simulink model "Progetto_1_0"  (R2015b)
settings: Solver=FixedStepDiscrete  SolverMode=SingleTasking  StartTime=0.0  StopTime=1500  FixedStep=1/100  RelTol=1e-3
values from neighbouring files (symbols this model uses):
  End_Time = s*z + l*z + l*x + 10    [Start_1_0.m]
  MASK = [0.111111111111  0.111111111111  0.111111111111; 0.111111111111  0.111111111111  0.111111111111; 0.111111111111  0.111111111111  0.111111111111]    [mask_3x3.mat]    (also in mask_3x3_egual.mat = [0  0  0; 0  1  0; 0  0  0]; mask_3x3_zeros.mat = [0  0  0; 0  0  0; 0  0  0]; mask_5x5.mat = [0.04 0.04 0.04 0.04 0.04 0.04 0.04 0.04 0.04 0.04 0.04 0.04; mask_5x5_egual.mat = [0 0 0 0 0 0 0 0 0 0 0 0 ... (25 elements, 5x5)])
libraries: hdlsllib x3, visionsources x1
settings Model: Creator=danilo  LastModifiedBy=danilo

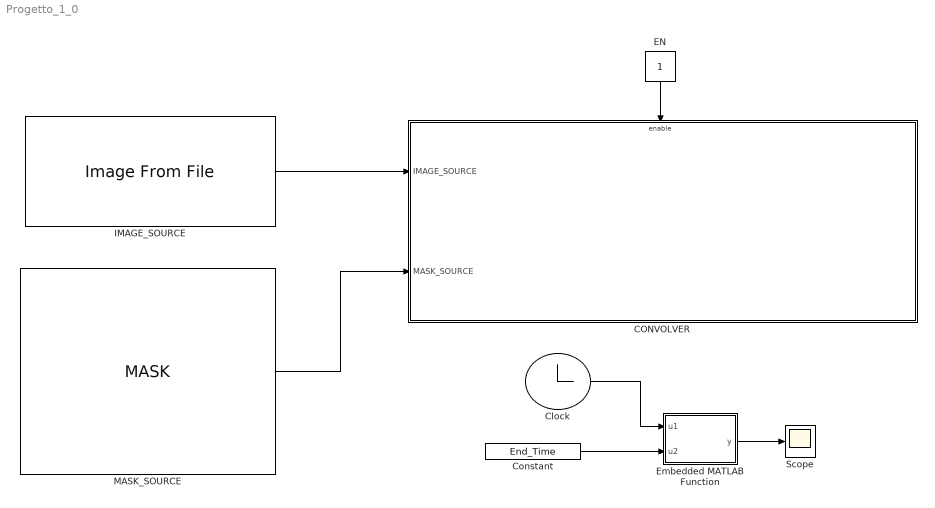
== system Progetto_1_0 ==
  CONVOLVER : Subsystem
  Clock : Clock
  Constant : Constant  Value=End_Time
  EN : Constant
  Embedded MATLAB Function : MATLAB Function  TreatAsAtomicUnit=on
  IMAGE_SOURCE : visionsources/Image From File  Tag=vipblks_nd  FileName=./test_23x10.jpg  imagePorts=One multidimensional signal  Ts=inf  ImageDataType=Inherit from input image  Signed=on  WordLength=16  sdImageDataType=uint(8)  FractionLengthMode=User-defined  FractionLength=15  OutPortLabels=R|G|B
  "MASK_SOURCE " : Constant  Value=MASK
  Scope : Scope
  wires:
  IMAGE_SOURCE/1 -> CONVOLVER/1(IMAGE_SOURCE)
  EN/1 -> CONVOLVER/Enable
  Clock/1 -> Embedded MATLAB Function/1(u1)
  Constant/1 -> Embedded MATLAB Function/2(u2)
  Embedded MATLAB Function/1(y) -> Scope/1
  "MASK_SOURCE "/1 -> CONVOLVER/2(MASK_SOURCE)

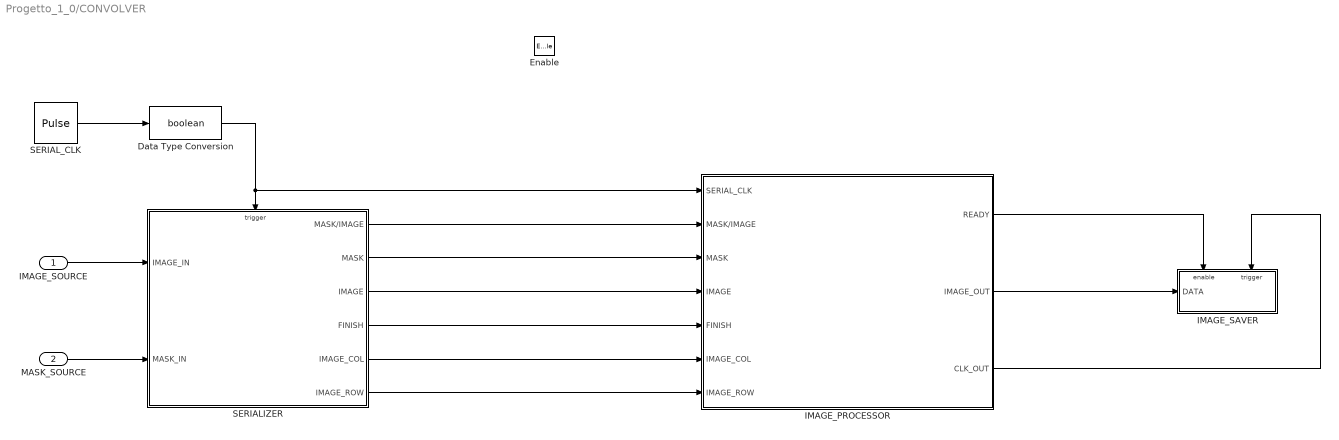
== system Progetto_1_0/CONVOLVER ==
  IMAGE_SOURCE : Inport
  MASK_SOURCE : Inport  Port=2
  Enable : EnablePort
  Data Type Conversion : DataTypeConversion  OutDataTypeStr=boolean
  IMAGE_PROCESSOR : Subsystem
  "IMAGE_SAVER " : Subsystem  TreatAsAtomicUnit=on
  SERIALIZER : Subsystem
  SERIAL_CLK : DiscretePulseGenerator  PulseType=Time based  Period=1  PulseWidth=50
  wires:
  MASK_SOURCE/1 -> SERIALIZER/2(MASK_IN)
  IMAGE_SOURCE/1 -> SERIALIZER/1(IMAGE_IN)
  SERIALIZER/5(IMAGE_COL) -> IMAGE_PROCESSOR/6(IMAGE_COL)
  SERIALIZER/3(IMAGE) -> IMAGE_PROCESSOR/4(IMAGE)
  SERIALIZER/4(FINISH) -> IMAGE_PROCESSOR/5(FINISH)
  SERIAL_CLK/1 -> Data Type Conversion/1
  Data Type Conversion/1 -> IMAGE_PROCESSOR/1(SERIAL_CLK), SERIALIZER/Trigger
  SERIALIZER/2(MASK) -> IMAGE_PROCESSOR/3(MASK)
  SERIALIZER/1(MASK/IMAGE) -> IMAGE_PROCESSOR/2(MASK/IMAGE)
  SERIALIZER/6(IMAGE_ROW) -> IMAGE_PROCESSOR/7(IMAGE_ROW)
  IMAGE_PROCESSOR/2(IMAGE_OUT) -> "IMAGE_SAVER "/1(DATA)
  IMAGE_PROCESSOR/1(READY) -> "IMAGE_SAVER "/Enable
  IMAGE_PROCESSOR/3(CLK_OUT) -> "IMAGE_SAVER "/Trigger

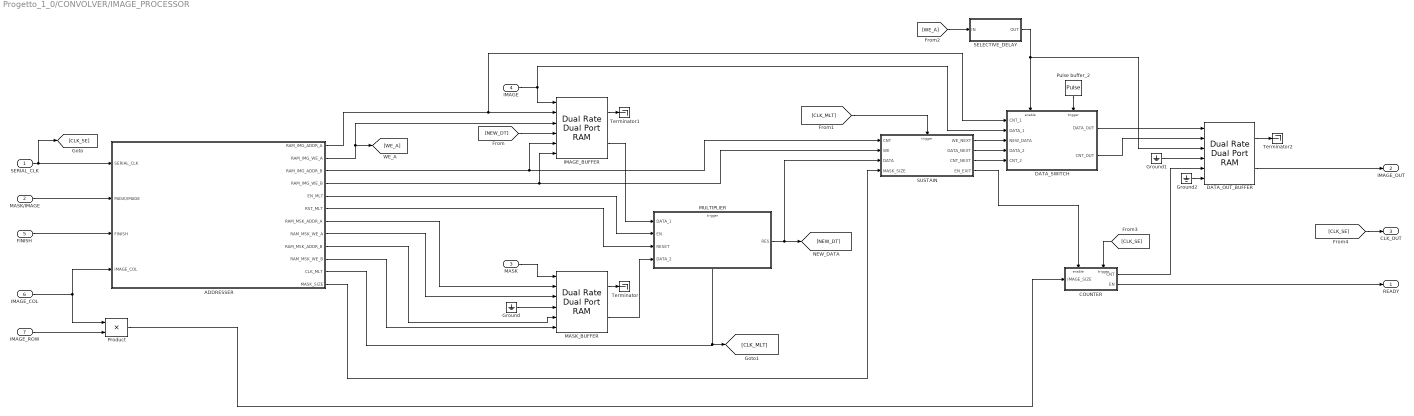
== system Progetto_1_0/CONVOLVER/IMAGE_PROCESSOR ==
  SERIAL_CLK : Inport  OutDataTypeStr=boolean
  MASK/IMAGE : Inport  Port=2  OutDataTypeStr=boolean
  MASK : Inport  Port=3  OutDataTypeStr=double
  IMAGE : Inport  Port=4  OutDataTypeStr=uint8
  FINISH : Inport  Port=5  OutDataTypeStr=boolean
  IMAGE_COL : Inport  Port=6  OutDataTypeStr=double
  IMAGE_ROW : Inport  Port=7  OutDataTypeStr=double
  ADDRESSER : Subsystem  TreatAsAtomicUnit=on
  COUNTER : Subsystem  TreatAsAtomicUnit=on
  DATA_OUT_BUFFER : hdlsllib/HDL Operations/Dual Rate Dual Port RAM  ram_size=16
  DATA_SWITCH : Subsystem  TreatAsAtomicUnit=on
  Ground : Ground
  Ground1 : Ground
  Ground2 : Ground
  IMAGE_BUFFER : hdlsllib/HDL Operations/Dual Rate Dual Port RAM  ram_size=16
  MASK_BUFFER : hdlsllib/HDL Operations/Dual Rate Dual Port RAM  ram_size=16
  MULTIPLIER : Subsystem
  Product : Product
  "Pulse buffer_2 " : DiscretePulseGenerator  PulseType=Time based  Period=1/2  PulseWidth=50
  SELECTIVE_DELAY : Subsystem
  SUSTAIN : Subsystem  TreatAsAtomicUnit=on
  Terminator : Terminator
  Terminator1 : Terminator
  Terminator2 : Terminator
  READY : Outport
  IMAGE_OUT : Outport  Port=2
  CLK_OUT : Outport  Port=3
  wires:
  MASK/IMAGE/1 -> ADDRESSER/2(MASK/IMAGE)
  MASK/1 -> MASK_BUFFER/1
  IMAGE/1 -> IMAGE_BUFFER/1, DATA_SWITCH/2(DATA_1)
  ADDRESSER/3(RAM_IMG_ADDR_B) -> SUSTAIN/1(CNT), IMAGE_BUFFER/5
  ADDRESSER/7(RAM_MSK_ADDR_A) -> MASK_BUFFER/2
  ADDRESSER/8("RAM_MSK_WE_A ") -> MASK_BUFFER/3
  ADDRESSER/9(RAM_MSK_ADDR_B) -> MASK_BUFFER/5
  ADDRESSER/10(RAM_MSK_WE_B) -> MASK_BUFFER/6
  MASK_BUFFER/2 -> MULTIPLIER/4(DATA_2)
  ADDRESSER/5(EN_MLT) -> MULTIPLIER/2(EN)
  ADDRESSER/6(RST_MLT) -> MULTIPLIER/3(RESET)
  MULTIPLIER/1(RES) -> SUSTAIN/3(DATA), [NEW_DT]
  [NEW_DT] -> IMAGE_BUFFER/4
  IMAGE_COL/1 -> Product/1, ADDRESSER/4(IMAGE_COL)
  ADDRESSER/11(CLK_MLT) -> [CLK_MLT], MULTIPLIER/Trigger
  MASK_BUFFER/1 -> Terminator/1
  Ground/1 -> MASK_BUFFER/4
  IMAGE_BUFFER/2 -> MULTIPLIER/1(DATA_1)
  "Pulse buffer_2 "/1 -> DATA_SWITCH/Trigger
  ADDRESSER/2("RAM_IMG_WE_A ") -> [WE_A], IMAGE_BUFFER/3
  SERIAL_CLK/1 -> [CLK_SE], ADDRESSER/1(SERIAL_CLK)
  SUSTAIN/2(DATA_NEXT) -> DATA_SWITCH/4(DATA_2)
  SUSTAIN/1(WE_NEXT) -> DATA_SWITCH/3(NEW_DATA)
  DATA_SWITCH/2(CNT_OUT) -> DATA_OUT_BUFFER/2
  DATA_OUT_BUFFER/2 -> IMAGE_OUT/1
  [WE_A] -> SELECTIVE_DELAY/1(IN)
  SELECTIVE_DELAY/1(OUT) -> DATA_SWITCH/Enable, DATA_OUT_BUFFER/3
  ADDRESSER/1(RAM_IMG_ADDR_A) -> DATA_SWITCH/1(CNT_1), IMAGE_BUFFER/2
  [CLK_SE] -> COUNTER/Trigger
  COUNTER/1(CNT) -> DATA_OUT_BUFFER/5
  FINISH/1 -> ADDRESSER/3(FINISH)
  DATA_SWITCH/1(DATA_OUT) -> DATA_OUT_BUFFER/1
  ADDRESSER/4(RAM_IMG_WE_B) -> SUSTAIN/2(WE), IMAGE_BUFFER/6
  SUSTAIN/3(CNT_NEXT) -> DATA_SWITCH/5(CNT_2)
  SUSTAIN/4(EN_EXIT) -> COUNTER/Enable
  [CLK_MLT] -> SUSTAIN/Trigger
  ADDRESSER/12(MASK_SIZE) -> SUSTAIN/4(MASK_SIZE)
  IMAGE_BUFFER/1 -> Terminator1/1
  Ground1/1 -> DATA_OUT_BUFFER/4
  Ground2/1 -> DATA_OUT_BUFFER/6
  IMAGE_ROW/1 -> Product/2
  Product/1 -> COUNTER/1(IMAGE_SIZE)
  COUNTER/2(EN) -> READY/1
  [CLK_SE] -> CLK_OUT/1
  DATA_OUT_BUFFER/1 -> Terminator2/1

== system Progetto_1_0/CONVOLVER/IMAGE_SAVER  ==
  DATA : Inport
  Enable : EnablePort
  Trigger : TriggerPort
  To Workspace : ToWorkspace  VariableName=simout  SampleTime=-1
      settings: Save2DSignal=2-D array (concatenate along first dimension)
  wires:
  DATA/1 -> To Workspace/1

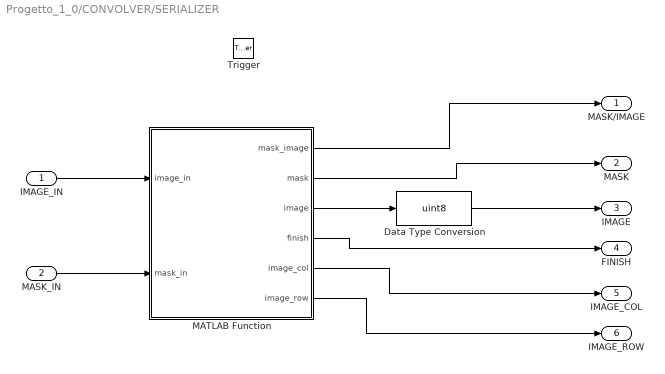
== system Progetto_1_0/CONVOLVER/SERIALIZER ==
  IMAGE_IN : Inport  OutDataTypeStr=uint8
  MASK_IN : Inport  Port=2
  Trigger : TriggerPort  PortDimensions=1
  Data Type Conversion : DataTypeConversion  OutDataTypeStr=uint8
  MATLAB Function : MATLAB Function  TreatAsAtomicUnit=on
  MASK/IMAGE : Outport
  MASK : Outport  Port=2  OutDataTypeStr=double
  IMAGE : Outport  Port=3
  FINISH : Outport  Port=4
  IMAGE_COL : Outport  Port=5  OutDataTypeStr=double
  IMAGE_ROW : Outport  Port=6  OutDataTypeStr=double
  wires:
  IMAGE_IN/1 -> MATLAB Function/1(image_in)
  MASK_IN/1 -> MATLAB Function/2(mask_in)
  MATLAB Function/1(mask_image) -> MASK/IMAGE/1
  MATLAB Function/3(image) -> Data Type Conversion/1
  MATLAB Function/4(finish) -> FINISH/1
  MATLAB Function/2(mask) -> MASK/1
  Data Type Conversion/1 -> IMAGE/1
  MATLAB Function/5(image_col) -> IMAGE_COL/1
  MATLAB Function/6(image_row) -> IMAGE_ROW/1

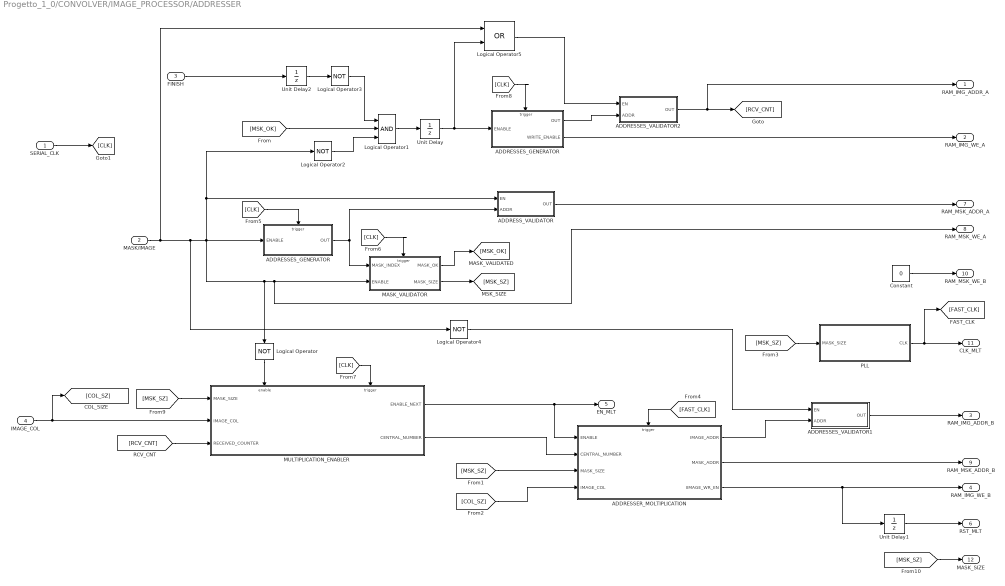
== system Progetto_1_0/CONVOLVER/IMAGE_PROCESSOR/ADDRESSER ==
  SERIAL_CLK : Inport
  MASK/IMAGE : Inport  Port=2
  FINISH : Inport  Port=3
  IMAGE_COL : Inport  Port=4  OutDataTypeStr=double
  ADDRESSER_MOLTIPLICATION : Subsystem  TreatAsAtomicUnit=on
  ADDRESSES_GENERATOR : Subsystem
  "ADDRESSES_GENERATOR " : Subsystem
  ADDRESSES_VALIDATOR1 : Subsystem
  ADDRESSES_VALIDATOR2 : Subsystem
  ADDRESS_VALIDATOR : Subsystem
  Constant : Constant  Value=0  OutDataTypeStr=boolean
  Logical Operator{,2..4} (4 alike) : Logic  Operator=NOT  AllPortsSameDT=off  OutDataTypeStr=boolean
  Logical Operator1 : Logic  Inputs=3  AllPortsSameDT=off  OutDataTypeStr=boolean
  Logical Operator5 : Logic  Operator=OR  AllPortsSameDT=off  OutDataTypeStr=boolean
  MASK_VALIDATOR : Subsystem
  MULTIPLICATION_ENABLER : Subsystem  TreatAsAtomicUnit=on
  PLL : Subsystem  TreatAsAtomicUnit=on
  Unit Delay : UnitDelay  SampleTime=-1
  Unit Delay1 : UnitDelay  SampleTime=-1
  Unit Delay2 : UnitDelay  SampleTime=-1
  RAM_IMG_ADDR_A : Outport
  "RAM_IMG_WE_A " : Outport  Port=2
  RAM_IMG_ADDR_B : Outport  Port=3
  RAM_IMG_WE_B : Outport  Port=4
  EN_MLT : Outport  Port=5
  RST_MLT : Outport  Port=6
  RAM_MSK_ADDR_A : Outport  Port=7  OutDataTypeStr=uint16
  "RAM_MSK_WE_A " : Outport  Port=8
  RAM_MSK_ADDR_B : Outport  Port=9
  RAM_MSK_WE_B : Outport  Port=10
  CLK_MLT : Outport  Port=11
  MASK_SIZE : Outport  Port=12
  wires:
  "ADDRESSES_GENERATOR "/1(OUT) -> ADDRESS_VALIDATOR/2(ADDR), MASK_VALIDATOR/1(MASK_INDEX)
  MASK_VALIDATOR/1(MASK_OK) -> [MSK_OK]
  Logical Operator1/1 -> Unit Delay/1
  Unit Delay/1 -> Logical Operator5/2, ADDRESSES_GENERATOR/1(ENABLE)
  FINISH/1 -> Unit Delay2/1
  ADDRESSES_VALIDATOR1/1(OUT) -> RAM_IMG_ADDR_B/1
  IMAGE_COL/1 -> MULTIPLICATION_ENABLER/2(IMAGE_COL), [COL_SZ]
  [RCV_CNT] -> MULTIPLICATION_ENABLER/3(RECEIVED_COUNTER)
  Logical Operator/1 -> MULTIPLICATION_ENABLER/Enable
  MULTIPLICATION_ENABLER/2(CENTRAL_NUMBER) -> ADDRESSER_MOLTIPLICATION/2(CENTRAL_NUMBER)
  [MSK_SZ] -> ADDRESSER_MOLTIPLICATION/3(MASK_SIZE)
  [COL_SZ] -> ADDRESSER_MOLTIPLICATION/4(IMAGE_COL)
  ADDRESSER_MOLTIPLICATION/1(IMAGE_ADDR) -> ADDRESSES_VALIDATOR1/2(ADDR)
  ADDRESSER_MOLTIPLICATION/2(MASK_ADDR) -> RAM_MSK_ADDR_B/1
  Constant/1 -> RAM_MSK_WE_B/1
  Unit Delay1/1 -> RST_MLT/1
  PLL/1(CLK) -> [FAST_CLK], CLK_MLT/1
  [MSK_SZ] -> PLL/1(MASK_SIZE)
  [FAST_CLK] -> ADDRESSER_MOLTIPLICATION/Trigger
  SERIAL_CLK/1 -> [CLK]
  [CLK] -> "ADDRESSES_GENERATOR "/Trigger
  [CLK] -> MASK_VALIDATOR/Trigger
  [CLK] -> MULTIPLICATION_ENABLER/Trigger
  [CLK] -> ADDRESSES_GENERATOR/Trigger
  ADDRESS_VALIDATOR/1(OUT) -> RAM_MSK_ADDR_A/1
  MASK_VALIDATOR/2(MASK_SIZE) -> [MSK_SZ]
  [MSK_SZ] -> MULTIPLICATION_ENABLER/1(MASK_SIZE)
  Unit Delay2/1 -> Logical Operator3/1
  ADDRESSES_GENERATOR/2(WRITE_ENABLE) -> "RAM_IMG_WE_A "/1
  ADDRESSER_MOLTIPLICATION/3(IIMAGE_WR_EN) -> Unit Delay1/1, RAM_IMG_WE_B/1
  Logical Operator2/1 -> Logical Operator1/3
  [MSK_OK] -> Logical Operator1/2
  Logical Operator3/1 -> Logical Operator1/1
  MULTIPLICATION_ENABLER/1("ENABLE_NEXT ") -> ADDRESSER_MOLTIPLICATION/1(ENABLE), EN_MLT/1
  Logical Operator4/1 -> ADDRESSES_VALIDATOR1/1(EN)
  MASK/IMAGE/1 -> "ADDRESSES_GENERATOR "/1(ENABLE), Logical Operator/1, "RAM_MSK_WE_A "/1, MASK_VALIDATOR/2(ENABLE), ADDRESS_VALIDATOR/1(EN), Logical Operator2/1, Logical Operator4/1, Logical Operator5/1
  ADDRESSES_VALIDATOR2/1(OUT) -> RAM_IMG_ADDR_A/1, [RCV_CNT]
  ADDRESSES_GENERATOR/1(OUT) -> ADDRESSES_VALIDATOR2/2(ADDR)
  Logical Operator5/1 -> ADDRESSES_VALIDATOR2/1(EN)
  [MSK_SZ] -> MASK_SIZE/1

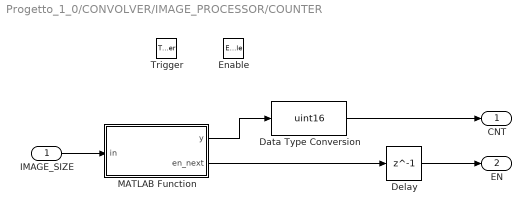
== system Progetto_1_0/CONVOLVER/IMAGE_PROCESSOR/COUNTER ==
  IMAGE_SIZE : Inport
  Enable : EnablePort
  Trigger : TriggerPort
  Data Type Conversion : DataTypeConversion  OutDataTypeStr=uint16
  Delay : Delay  DelayLength=1  InitialCondition=0
  MATLAB Function : MATLAB Function  TreatAsAtomicUnit=on
  CNT : Outport
  EN : Outport  Port=2
  wires:
  MATLAB Function/1(y) -> Data Type Conversion/1
  Data Type Conversion/1 -> CNT/1
  IMAGE_SIZE/1 -> MATLAB Function/1(in)
  MATLAB Function/2(en_next) -> Delay/1
  Delay/1 -> EN/1

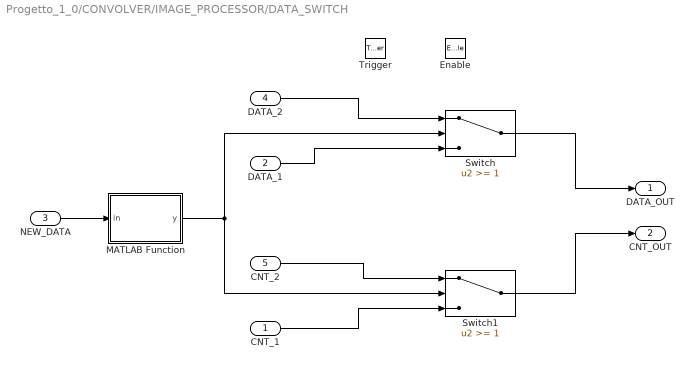
== system Progetto_1_0/CONVOLVER/IMAGE_PROCESSOR/DATA_SWITCH ==
  CNT_1 : Inport
  DATA_1 : Inport  Port=2
  NEW_DATA : Inport  Port=3
  DATA_2 : Inport  Port=4
  CNT_2 : Inport  Port=5
  Enable : EnablePort
  Trigger : TriggerPort
  MATLAB Function : MATLAB Function  TreatAsAtomicUnit=on
  Switch : Switch  Threshold=1
  Switch1 : Switch  Threshold=1
  DATA_OUT : Outport
  CNT_OUT : Outport  Port=2
  wires:
  Switch/1 -> DATA_OUT/1
  DATA_2/1 -> Switch/1
  DATA_1/1 -> Switch/3
  CNT_2/1 -> Switch1/1
  Switch1/1 -> CNT_OUT/1
  CNT_1/1 -> Switch1/3
  NEW_DATA/1 -> MATLAB Function/1(in)
  MATLAB Function/1(y) -> Switch/2, Switch1/2

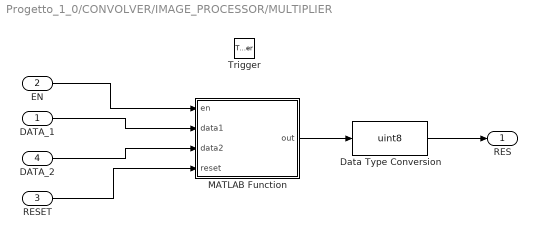
== system Progetto_1_0/CONVOLVER/IMAGE_PROCESSOR/MULTIPLIER ==
  DATA_1 : Inport
  EN : Inport  Port=2
  RESET : Inport  Port=3
  DATA_2 : Inport  Port=4
  Trigger : TriggerPort  PortDimensions=1
  Data Type Conversion : DataTypeConversion  OutDataTypeStr=uint8
  MATLAB Function : MATLAB Function  TreatAsAtomicUnit=on
  RES : Outport
  wires:
  MATLAB Function/1(out) -> Data Type Conversion/1
  EN/1 -> MATLAB Function/1(en)
  DATA_1/1 -> MATLAB Function/2(data1)
  DATA_2/1 -> MATLAB Function/3(data2)
  Data Type Conversion/1 -> RES/1
  RESET/1 -> MATLAB Function/4(reset)

== system Progetto_1_0/CONVOLVER/IMAGE_PROCESSOR/SELECTIVE_DELAY ==
  IN : Inport
  Switch : Switch  Threshold=1
  Unit Delay : UnitDelay  SampleTime=-1
  OUT : Outport
  wires:
  Unit Delay/1 -> Switch/3
  Switch/1 -> OUT/1
  IN/1 -> Unit Delay/1, Switch/1, Switch/2

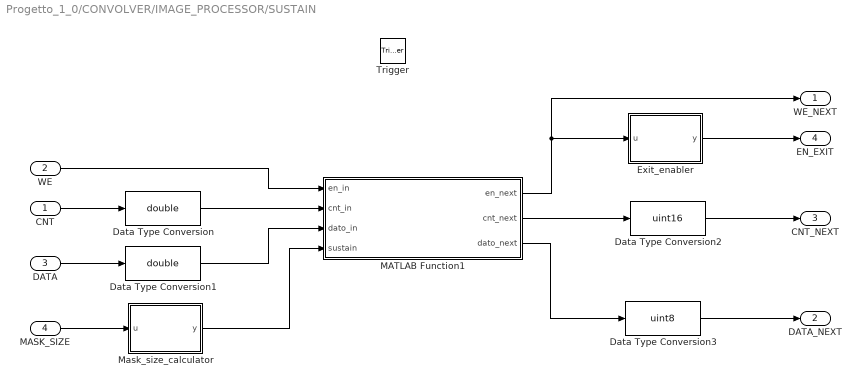
== system Progetto_1_0/CONVOLVER/IMAGE_PROCESSOR/SUSTAIN ==
  CNT : Inport
  WE : Inport  Port=2
  DATA : Inport  Port=3
  MASK_SIZE : Inport  Port=4
  Trigger : TriggerPort
  Data Type Conversion : DataTypeConversion  OutDataTypeStr=double
  Data Type Conversion1 : DataTypeConversion  OutDataTypeStr=double
  Data Type Conversion2 : DataTypeConversion  OutDataTypeStr=uint16
  Data Type Conversion3 : DataTypeConversion  OutDataTypeStr=uint8
  Exit_enabler : MATLAB Function  TreatAsAtomicUnit=on
  MATLAB Function1 : MATLAB Function  TreatAsAtomicUnit=on
  Mask_size_calculator : MATLAB Function  TreatAsAtomicUnit=on
  WE_NEXT : Outport
  DATA_NEXT : Outport  Port=2
  CNT_NEXT : Outport  Port=3
  EN_EXIT : Outport  Port=4
  wires:
  Exit_enabler/1(y) -> EN_EXIT/1
  WE/1 -> MATLAB Function1/1(en_in)
  MATLAB Function1/2(cnt_next) -> Data Type Conversion2/1
  MATLAB Function1/1(en_next) -> Exit_enabler/1(u), WE_NEXT/1
  MATLAB Function1/3(dato_next) -> Data Type Conversion3/1
  DATA/1 -> Data Type Conversion1/1
  CNT/1 -> Data Type Conversion/1
  Data Type Conversion/1 -> MATLAB Function1/2(cnt_in)
  Data Type Conversion1/1 -> MATLAB Function1/3(dato_in)
  Data Type Conversion2/1 -> CNT_NEXT/1
  Data Type Conversion3/1 -> DATA_NEXT/1
  MASK_SIZE/1 -> Mask_size_calculator/1(u)
  Mask_size_calculator/1(y) -> MATLAB Function1/4(sustain)

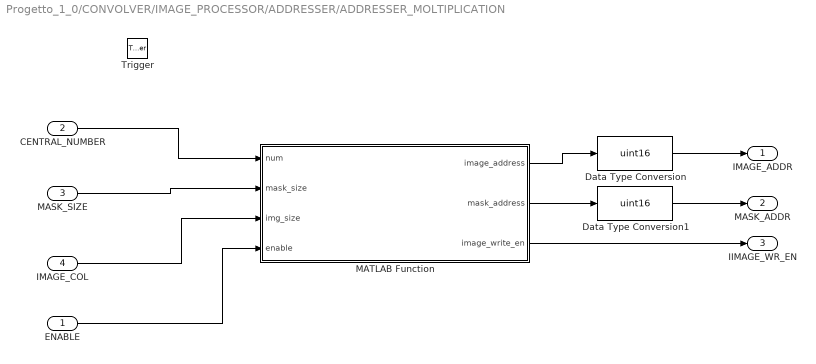
== system Progetto_1_0/CONVOLVER/IMAGE_PROCESSOR/ADDRESSER/ADDRESSER_MOLTIPLICATION ==
  ENABLE : Inport
  CENTRAL_NUMBER : Inport  Port=2
  MASK_SIZE : Inport  Port=3
  IMAGE_COL : Inport  Port=4
  Trigger : TriggerPort
  Data Type Conversion : DataTypeConversion  OutDataTypeStr=uint16
  Data Type Conversion1 : DataTypeConversion  OutDataTypeStr=uint16
  MATLAB Function : MATLAB Function  TreatAsAtomicUnit=on
  IMAGE_ADDR : Outport
  MASK_ADDR : Outport  Port=2
  IIMAGE_WR_EN : Outport  Port=3
  wires:
  CENTRAL_NUMBER/1 -> MATLAB Function/1(num)
  MASK_SIZE/1 -> MATLAB Function/2(mask_size)
  IMAGE_COL/1 -> MATLAB Function/3(img_size)
  MATLAB Function/1(image_address) -> Data Type Conversion/1
  MATLAB Function/2(mask_address) -> Data Type Conversion1/1
  MATLAB Function/3(image_write_en) -> IIMAGE_WR_EN/1
  Data Type Conversion/1 -> IMAGE_ADDR/1
  Data Type Conversion1/1 -> MASK_ADDR/1
  ENABLE/1 -> MATLAB Function/4(enable)

== system Progetto_1_0/CONVOLVER/IMAGE_PROCESSOR/ADDRESSER/ADDRESSES_GENERATOR ==
  ENABLE : Inport
  Trigger : TriggerPort  PortDimensions=1
  Data Type Conversion : DataTypeConversion  OutDataTypeStr=uint16
  MATLAB Function : MATLAB Function  TreatAsAtomicUnit=on
  OUT : Outport  OutDataTypeStr=uint16
  WRITE_ENABLE : Outport  Port=2  OutDataTypeStr=boolean
  wires:
  ENABLE/1 -> MATLAB Function/1(enable)
  MATLAB Function/1(out) -> Data Type Conversion/1
  Data Type Conversion/1 -> OUT/1
  MATLAB Function/2(write_en) -> WRITE_ENABLE/1

== system Progetto_1_0/CONVOLVER/IMAGE_PROCESSOR/ADDRESSER/ADDRESSES_GENERATOR  ==
  ENABLE : Inport
  Trigger : TriggerPort  PortDimensions=1
  Data Type Conversion : DataTypeConversion  OutDataTypeStr=uint16
  MATLAB Function : MATLAB Function  TreatAsAtomicUnit=on
  OUT : Outport  OutDataTypeStr=uint16
  wires:
  ENABLE/1 -> MATLAB Function/1(enable)
  MATLAB Function/1(out) -> Data Type Conversion/1
  Data Type Conversion/1 -> OUT/1

== system Progetto_1_0/CONVOLVER/IMAGE_PROCESSOR/ADDRESSER/ADDRESSES_VALIDATOR1 ==
  EN : Inport
  ADDR : Inport  Port=2
  Constant : Constant  Value=65000  OutDataTypeStr=uint16
  Switch : Switch  Threshold=1  OutDataTypeStr=uint16
  OUT : Outport  OutDataTypeStr=uint16
  wires:
  EN/1 -> Switch/2
  ADDR/1 -> Switch/1
  Switch/1 -> OUT/1
  Constant/1 -> Switch/3

== system Progetto_1_0/CONVOLVER/IMAGE_PROCESSOR/ADDRESSER/ADDRESSES_VALIDATOR2 ==
  EN : Inport
  ADDR : Inport  Port=2
  Constant : Constant  Value=65000  OutDataTypeStr=uint16
  Switch : Switch  Threshold=1  OutDataTypeStr=uint16
  OUT : Outport
  wires:
  EN/1 -> Switch/2
  ADDR/1 -> Switch/1
  Switch/1 -> OUT/1
  Constant/1 -> Switch/3

== system Progetto_1_0/CONVOLVER/IMAGE_PROCESSOR/ADDRESSER/ADDRESS_VALIDATOR ==
  EN : Inport
  ADDR : Inport  Port=2
  Constant : Constant  Value=65000  OutDataTypeStr=uint16
  Switch : Switch  Threshold=1  OutDataTypeStr=uint16
  OUT : Outport
  wires:
  EN/1 -> Switch/2
  ADDR/1 -> Switch/1
  Switch/1 -> OUT/1
  Constant/1 -> Switch/3

== system Progetto_1_0/CONVOLVER/IMAGE_PROCESSOR/ADDRESSER/MASK_VALIDATOR ==
  MASK_INDEX : Inport
  ENABLE : Inport  Port=2
  Trigger : TriggerPort  PortDimensions=1
  MATLAB Function : MATLAB Function  TreatAsAtomicUnit=on
  MASK_OK : Outport
  MASK_SIZE : Outport  Port=2
  wires:
  ENABLE/1 -> MATLAB Function/2(enable)
  MATLAB Function/1(mask_ok) -> MASK_OK/1
  MASK_INDEX/1 -> MATLAB Function/1(mask_in)
  MATLAB Function/2(mask_size) -> MASK_SIZE/1

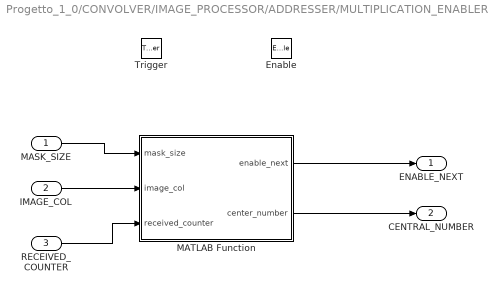
== system Progetto_1_0/CONVOLVER/IMAGE_PROCESSOR/ADDRESSER/MULTIPLICATION_ENABLER ==
  MASK_SIZE : Inport
  IMAGE_COL : Inport  Port=2
  RECEIVED_COUNTER : Inport  Port=3
  Enable : EnablePort
  Trigger : TriggerPort
  MATLAB Function : MATLAB Function  TreatAsAtomicUnit=on
  "ENABLE_NEXT " : Outport
  CENTRAL_NUMBER : Outport  Port=2
  wires:
  IMAGE_COL/1 -> MATLAB Function/2(image_col)
  MASK_SIZE/1 -> MATLAB Function/1(mask_size)
  RECEIVED_COUNTER/1 -> MATLAB Function/3(received_counter)
  MATLAB Function/1(enable_next) -> "ENABLE_NEXT "/1
  MATLAB Function/2(center_number) -> CENTRAL_NUMBER/1

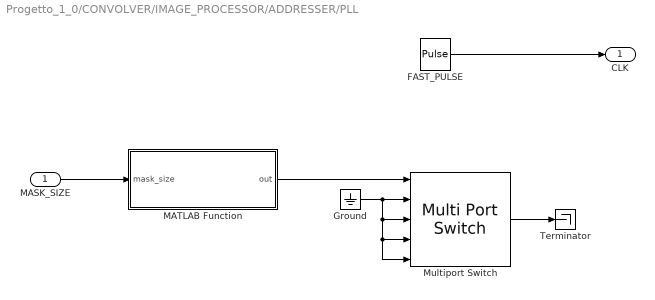
== system Progetto_1_0/CONVOLVER/IMAGE_PROCESSOR/ADDRESSER/PLL ==
  MASK_SIZE : Inport
  FAST_PULSE : DiscretePulseGenerator  PulseType=Time based  Period=1/50  PulseWidth=50
  Ground : Ground
  MATLAB Function : MATLAB Function  TreatAsAtomicUnit=on
  Multiport Switch : MultiPortSwitch  Inputs=4
  Terminator : Terminator
  CLK : Outport
  wires:
  MASK_SIZE/1 -> MATLAB Function/1(mask_size)
  MATLAB Function/1(out) -> Multiport Switch/1
  FAST_PULSE/1 -> CLK/1
  Multiport Switch/1 -> Terminator/1
  Ground/1 -> Multiport Switch/5, Multiport Switch/4, Multiport Switch/3, Multiport Switch/2

== matlab function Progetto_1_0/CONVOLVER/IMAGE_PROCESSOR/ADDRESSER/ADDRESSER_MOLTIPLICATION/MATLAB Function ==
  data: num input; image_address output; mask_size input; img_size input; mask_address output; image_write_en output; enable input
function [image_address, mask_address, image_write_en] = fnc( num, mask_size, img_size, enable )

    persistent x;
    persistent index;
    persistent counter;
    persistent cnt_mask;
    
    if(enable == 1)                             %se il blocco è abilitato
        
            if(isempty(counter))                    %inizializzo le variabili
                counter = 0; 
            end
    
        if(isempty(x) || counter == 0)
            cnt_mask = 1;
            counter = 1;
            index = 0;
            x = (mask_size - 1) / 2;
            x = -x;
        end
        
        vect = 0;
                    
        if(mask_size == 3)                          %genero gli offset rispetto al baricantro per prelevare la sottomatrice
            vect = [-1 0 1];
        elseif(mask_size == 5)
            vect = [-2 -1 0 1 2];
        elseif(mask_size == 7)
            vect = [-3 -2 -1 0 1 2 3];
        end
        
        if(index == mask_size)
            x = x + 1;
            index = 0;
        end
    
        image_write_en = logical(false);
        
        if(counter == (mask_size^2 + 1))            %se ho finito di mandare tutti gli indirizzi, invio l'indirizzo del baricentro
                                                    %ed abilito write_enable
        
            image_address = num;
            image_write_en = logical(true);
            x = 0;
            index = 0;
            vect = 0;
            counter = 0;
            cnt_mask = 0;
        else                                        %altrimenti genero gli indirizzi
            
            image_address = num + (img_size * x) + vect(index + 1);
            index = index + 1;
            counter = counter + 1;
        end
    
        mask_address = cnt_mask;
        cnt_mask = cnt_mask + 1;
        
    else                                            %se il blocco è disabilitato 
        
        image_address = 0;
        mask_address = 0;
        image_write_en = logical(false);
    end
end

== matlab function Progetto_1_0/CONVOLVER/SERIALIZER/MATLAB Function ==
  data: image_in input; mask_image output; mask_in input; mask output; image output; finish output; image_col output; image_row output
function [mask_image, mask, image, finish, image_col, image_row] = fcn(image_in, mask_in)

    persistent status;                                  %variabile di stato mask/image
    persistent im_col;                                  %indice colonne immagine
    persistent im_row;                                  %indice righe immagine
    persistent msk_col;                                 %indice colonne maschera 
    persistent msk_row;                                 %indice righe maschera
    
    if(isempty(status))                                 %inizializzazione variabili
        status  = 1; 
        im_col  = 1;
        im_row  = 1;
        msk_col = 1;
        msk_row = 1;
    end
    
    [j, k] = size(image_in);            
    image_col = k;
    image_row = j;
    finish = logical(false);
    
    if(status == 1)                                     %se è abilitata la serializzazione della maschera
        
        [m, n] = size(mask_in);
        image = 0;
        
        if(msk_row > m)                                 %se sono finite le righe della maschera
            
            status = 2;                                 %setto lo stato per serializzare l'immagine
            mask = 0;
            mask_image = logical(false);    
        else                                            
                                                        %serializzo la maschera
            mask_image = logical(true)
            mask = mask_in(msk_row, msk_col);
            msk_col = msk_col + 1;
            
            if(msk_col > n)                             %vado a capo
                msk_col = 1;
                msk_row = msk_row + 1;
            end
        end
    else                                                %seriallizzazione immagine
       
        mask = 0;
        mask_image = logical(false);
        if(im_col > k)
            im_row = im_row + 1;
            im_col = 1;
        end
        
        if(im_row > j)                                  %se l'immagine è finita
            finish = logical(true);
            image = 0;
        else
            
            image = double(image_in(im_row, im_col));
            im_col = im_col + 1;
        end
    end
end

== matlab function Progetto_1_0/CONVOLVER/IMAGE_PROCESSOR/ADDRESSER/ADDRESSES_GENERATOR/MATLAB Function ==
  data: enable input; out output; write_en output
function [out, write_en] = fcn(enable)

    persistent cnt;                             %contatore
    persistent flag;            
    
    if(isempty(cnt))                            %inizializzazione
        cnt = 1;
        flag = 0;
    end
    
    if(enable == 1)                             %se il blocco è abilitato
        
        flag = 1;                               %flag = 1
        out = cnt;
        cnt = cnt + 1;
        write_en = logical(true);               %abilito la scrittura nella ram dell'immagine
    else                                        %se il blocco è disabilitato
        
        write_en = logical(false);          
        
        if(flag == 1)                           %la prima volta abilito il blocco successivo
            
            write_en = logical(true);
            flag = 0;                           %azzero flag
        end
        
        out = 0;            
    end
end

== matlab function Progetto_1_0/CONVOLVER/IMAGE_PROCESSOR/ADDRESSER/ADDRESSES_GENERATOR /MATLAB Function ==
  data: enable input; out output
function out = fcn(enable)

    persistent cnt;             %variabile contatore

    if(isempty(cnt))            %inizializzazione
    
        cnt = 1;
    end

    if(enable == 0)             %se il blocco è disabilitato
        
        out = 0; 
    else                        %altrimenti
        
        out = cnt;              
        cnt = cnt + 1;
    end

end

== matlab function Progetto_1_0/CONVOLVER/IMAGE_PROCESSOR/ADDRESSER/MULTIPLICATION_ENABLER/MATLAB Function ==
  data: mask_size input; enable_next output; image_col input; received_counter input; center_number output
function [ enable_next, center_number ] = fnc( mask_size, image_col, received_counter )

    persistent center_counter;                  %numero del baricentro
    persistent row;                                         %riga
    persistent dist;                                        %distanza
    
    spare = (mask_size - 1) / 2;                            %calcolo la dimensione dei bordi
    
    if(isempty(center_counter))
                                                            %inizializzo le variabili
        row = spare;                                        %mi posiziono nella riga che precede il primo baricentro
        center_counter = image_col*row + spare + 1;         %primo baricentro valido
        dist = center_counter;                              %distanza minima per poter effettuare le convoluzioni
        row = row + 1;                                      %incremento la riga
    end

    if(((received_counter - center_counter) == (dist)))     %se ho ricevuto un numero sufficiente di dati

        enable_next = logical(true);                        %abilito le moltiplicazioni
        center_number = center_counter;                     %setto l'uscita 
        center_counter = center_counter + 1;                %sposto il baricentro
        
        if(center_counter > (image_col * row - spare))      %se necessario sposto la riga e calcolo il nuovo baricentro
           
            row = row + 1;
            center_counter = center_counter + 2*spare; 
        end
    else                                                    %altrimenti aspetto di ricevere altri dati
       
        center_number = 0;
        enable_next = logical(false);
    end
    
    if(received_counter > (row + spare)*image_col + 1)      %se ho calcolato tutti i possibili baricentri, finisco
       
        center_number = 0;
        enable_next = logical(false);
    end
end

== matlab function Progetto_1_0/Embedded MATLAB Function ==
  settings: fimath=|
      | fimath(...
      | 'RoundMode', 'floor',...
      | 'OverflowMode', 'wrap',...
      | 'ProductMode', 'KeepLSB', 'ProductWordLength', 32,...
      | 'SumMode', 'KeepLSB', 'SumWordLength', 32,...
      | 'CastBeforeSum', false)
  data: u1 input; y output; u2 input
function y = fcn(u1, u2)
% This block supports an embeddable subset of the MATLAB language.
% See the help menu for details. 

coder.extrinsic('waitbar')
waitbar(u1/u2)
y = 1;

== matlab function Progetto_1_0/CONVOLVER/IMAGE_PROCESSOR/ADDRESSER/PLL/MATLAB Function ==
  data: mask_size input; out output
function out = fcn(mask_size)

    switch mask_size
       
        case 3
            out = 1;
        case 5
            out = 2;
        case 7
            out = 3;
        otherwise
            out = 4;
    end
end

== matlab function Progetto_1_0/CONVOLVER/IMAGE_PROCESSOR/MULTIPLIER/MATLAB Function ==
  data: out output; en input; data1 input; data2 input; reset input
function out = fcn(en, data1, data2, reset)

    persistent sum;                                 %variabile di stato per le somme parziali

    if(isempty(sum))                                %inizializzazione variabile
        
      sum = 0; 
    end
    
    if(reset == 1)                                  %se il reset è abilitato
        
       sum = 0; 
    end
    
    if(en == 0)                                     %se il blocco è disabilitato
        
        out = 0;
        sum = 0;
    else                                            %se il blocco è abilitato
        
       sum = double(sum + (data1*data2));           %somma parziale
    end
    
    out = sum;                                      %out = somma
end

== matlab function Progetto_1_0/CONVOLVER/IMAGE_PROCESSOR/COUNTER/MATLAB Function ==
  data: y output; in input; en_next output
function [y, en_next] = fcn(in)

    persistent cnt;                 %variabile contatore
    
    if(isempty(cnt))                %iniziallizzazione contatore
                        
       cnt = 1; 
    end
    
    if(cnt <= in)                   %se contatore è <= del numero di elementi dell'immagine
        
        y = cnt;                    
        cnt = cnt + 1;
        en_next = logical(true);    %abilito la seriale a ricevere i dati
    else
        
        en_next = logical(false);   %immagine finita
        y = 0; 
    end
end

== matlab function Progetto_1_0/CONVOLVER/IMAGE_PROCESSOR/ADDRESSER/MASK_VALIDATOR/MATLAB Function ==
  data: mask_in input; mask_ok output; enable input; mask_size output
function [mask_ok, mask_size] = fcn(mask_in, enable)

    persistent flag;                          
    persistent msk_size;
    
    if(isempty(flag))
        
        flag = logical(false);
        msk_size = 0;
    end
    
    if(enable == 1)                     %se il blocco è abilitato
        
        %se il numero di dati ricevuti è valido per la maschera
       if(sqrt(double(mask_in)) == 3 || sqrt(double(mask_in)) == 5 || sqrt(double(mask_in)) == 7)
           
           %abilito flag e salvo la dimensione della maschera
           flag = logical(true);
           msk_size = sqrt(double(mask_in));
       else
           
           flag = logical(false);
           
       end
    end
    
    mask_ok = flag;                     %il blocco successivo è abilitato se flag è uguale a uno
    mask_size = msk_size;               %mask_size conterrà la dimensione della maschera
    
end

== matlab function Progetto_1_0/CONVOLVER/IMAGE_PROCESSOR/DATA_SWITCH/MATLAB Function ==
  data: y output; in input
function y = fcn(in)

    persistent state;                   %variabile di stato
    
    if(isempty(state))                  %inizializzazione stato
        
       state = 0; 
    end
    
    y = 0;                              %uscita = 0
    
    if(state == 0 && in == 1)           
        
        state = 1;                      %stato = 1 
    else
        
        y = state;                      %l'uscita è abilitata se l'ingresso allo stato precedente era uno 
        state = 0;                      %riazzero lo stato
    end
end

== matlab function Progetto_1_0/CONVOLVER/IMAGE_PROCESSOR/SUSTAIN/Exit_enabler ==
  data: u input; y output
function y = fcn(u)
    
    persistent state;                       %variabile di stato
    
    if(isempty(state))                      %inizializzo la variabile
    
        state = logical(false); 
    end
    
    if(u == 1)                              %al primo ingresso alto abilito l'uscita dei dati
       
        state = logical(true);
    end
    
	y = state;
    
end

== matlab function Progetto_1_0/CONVOLVER/IMAGE_PROCESSOR/SUSTAIN/MATLAB Function1 ==
  data: en_in input; en_next output; cnt_in input; dato_in input; cnt_next output; dato_next output; sustain input
function [en_next, cnt_next, dato_next] = fcn(en_in, cnt_in, dato_in, sustain)

    persistent cnt;                                 %variabile contatore delle chiamate
    persistent state;                               %variabile che tiene conto se è stato scritto un dato in ram
    persistent dato_save;                           %dato inserito in ram
    persistent cnt_save;                            %indirizzo del dato
    
    if(isempty(state))                              %inizializzo le variabili
        
       state = logical(false); 
       cnt = 1;
       dato_save = 0;
       cnt_save = 0;
    end
    
    if(cnt == (sustain + 2))                        %se la funzione è stata chiamata un numero di volte per cui deve azzerarsi
        
        cnt = 1;
        state = logical(false);
        dato_save = 0;
        cnt_save = 0;
    end
    
    if(en_in == 1)                                  %se write_enable della ram è alto
        
        cnt = 1;                                    %mi sposto nello stato che mantiene i dati
        state = logical(true); 
        dato_save = dato_in;
        cnt_save = cnt_in;
    end
    
    if(state == 1)                                  %se sono nello stato di mantenimento incremento il contatore
        
        cnt = cnt + 1;
    end
    
    if(state == 1 && cnt > 2)                       %metto in uscita i dati salvati
        
        en_next = logical(true);
        cnt_next = cnt_save;
        dato_next = dato_save;
    else
        
        en_next = logical(false);                   %non devo mantenere alcun dato in uscita
        cnt_next = 0;
        dato_next = 0;
    end
    
end

== matlab function Progetto_1_0/CONVOLVER/IMAGE_PROCESSOR/SUSTAIN/Mask_size_calculator ==
  data: u input; y output
function y = fcn(u)
    
    %calcolo la frequenza del clock del moltiplicatore
    y= u^2 + 1;
    
end
